simulink model "Multiplier"  (R2019b)
settings: Solver=VariableStepAuto  StartTime=0.0  StopTime=10.0  RelTol=1e-3
libraries: hdlsllib x17
(part 1 of 3)
settings Model: Creator=cohen  LastModifiedBy=cohen

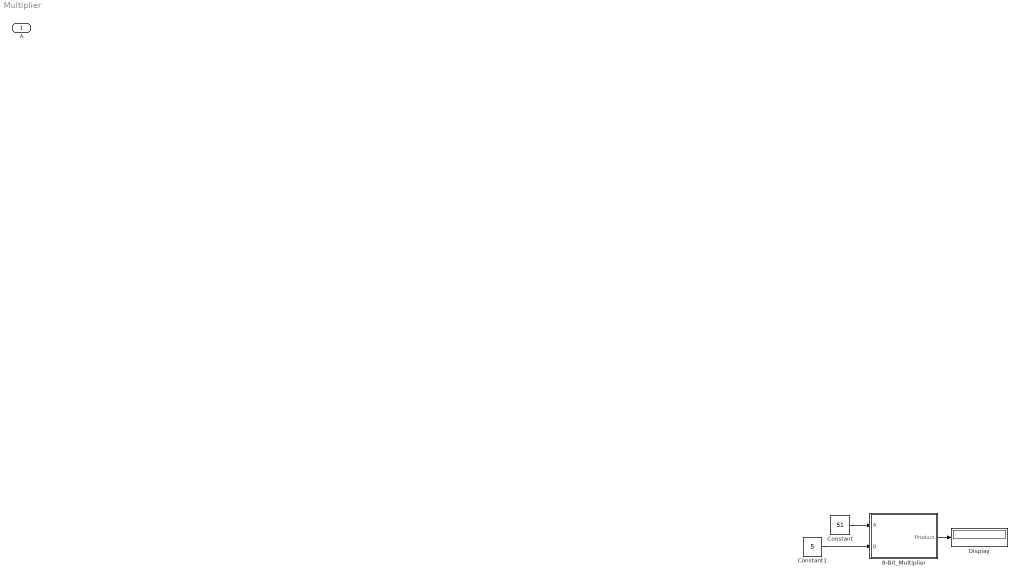
== system Multiplier ==
  A : Inport
  8-Bit_Multiplier : Subsystem
  Constant : Constant  Value=51  OutDataTypeStr=uint8
  Constant1 : Constant  Value=5  OutDataTypeStr=uint8
  Display : Display
  wires:
  8-Bit_Multiplier/1(Product) -> Display/1
  Constant/1 -> 8-Bit_Multiplier/1(A)
  Constant1/1 -> 8-Bit_Multiplier/2(B)

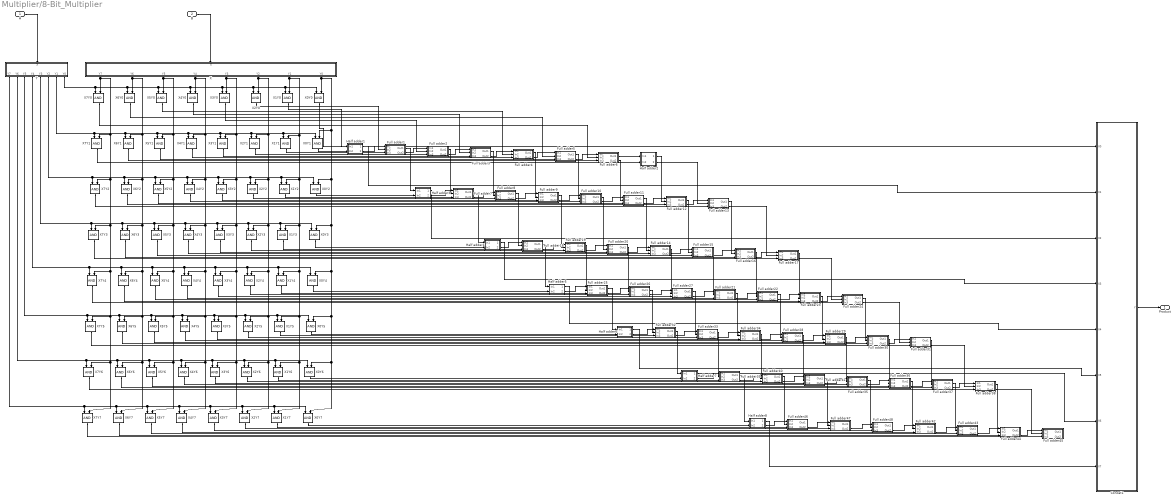
== system Multiplier/8-Bit_Multiplier ==
  A : Inport
  B : Inport  Port=2
  Concat1 : Subsystem
  Full adder1 : Subsystem
  Full adder10 : Subsystem
  Full adder11 : Subsystem
  Full adder12 : Subsystem
  Full adder13 : Subsystem
  Full adder14 : Subsystem
  Full adder15 : Subsystem
  Full adder16 : Subsystem
  Full adder17 : Subsystem
  Full adder18 : Subsystem
  Full adder19 : Subsystem
  Full adder2 : Subsystem
  Full adder20 : Subsystem
  Full adder21 : Subsystem
  Full adder22 : Subsystem
  Full adder23 : Subsystem
  Full adder24 : Subsystem
  Full adder25 : Subsystem
  Full adder26 : Subsystem
  Full adder27 : Subsystem
  Full adder28 : Subsystem
  Full adder29 : Subsystem
  Full adder3 : Subsystem
  Full adder30 : Subsystem
  Full adder31 : Subsystem
  Full adder32 : Subsystem
  Full adder33 : Subsystem
  Full adder34 : Subsystem
  Full adder35 : Subsystem
  Full adder36 : Subsystem
  Full adder37 : Subsystem
  Full adder38 : Subsystem
  Full adder39 : Subsystem
  Full adder4 : Subsystem
  Full adder40 : Subsystem
  Full adder41 : Subsystem
  Full adder42 : Subsystem
  Full adder43 : Subsystem
  Full adder44 : Subsystem
  Full adder45 : Subsystem
  Full adder46 : Subsystem
  Full adder47 : Subsystem
  Full adder48 : Subsystem
  Full adder5 : Subsystem
  Full adder6 : Subsystem
  Full adder7 : Subsystem
  Full adder8 : Subsystem
  Full adder9 : Subsystem
  Half adder1 : Subsystem
  Half adder2 : Subsystem
  Half adder3 : Subsystem
  Half adder4 : Subsystem
  Half adder5 : Subsystem
  Half adder6 : Subsystem
  Half adder7 : Subsystem
  Half adder8 : Subsystem
  X : Subsystem
  X0Y{0..7} (8 alike) : Logic  AllPortsSameDT=off  OutDataTypeStr=boolean
  X1Y{0..7} (8 alike) : Logic  AllPortsSameDT=off  OutDataTypeStr=boolean
  X2Y{0..7} (8 alike) : Logic  AllPortsSameDT=off  OutDataTypeStr=boolean
  X3Y{0..7} (8 alike) : Logic  AllPortsSameDT=off  OutDataTypeStr=boolean
  X4Y{0..7} (8 alike) : Logic  AllPortsSameDT=off  OutDataTypeStr=boolean
  X5Y{0..7} (8 alike) : Logic  AllPortsSameDT=off  OutDataTypeStr=boolean
  X6Y{0..7} (8 alike) : Logic  AllPortsSameDT=off  OutDataTypeStr=boolean
  X7Y{0..7} (8 alike) : Logic  AllPortsSameDT=off  OutDataTypeStr=boolean
  Y : Subsystem
  Product : Outport
  wires:
  X/3(Y5) -> X5Y1/2, X5Y7/2, X5Y6/2, X5Y5/2, X5Y4/2, X5Y3/2, X5Y2/2, X5Y0/2
  Full adder31/2(Out2) -> Full adder38/2(In2)
  Half adder5/1(Out1) -> Concat1/5(X4)
  Full adder4/1(Out1) -> Full adder9/2(In2)
  Full adder15/1(Out1) -> Full adder21/2(In2)
  Full adder10/2(Out2) -> Full adder11/1(In1)
  Full adder3/2(Out2) -> Full adder4/1(In1)
  Full adder7/2(Out2) -> Full adder8/1(In1)
  X/8(Y0) -> X0Y7/2, X0Y6/2, X0Y5/2, X0Y4/2, X0Y3/2, X0Y2/2, X0Y1/2, X0Y0/2
  Full adder21/2(Out2) -> Full adder22/1(In1)
  Full adder5/1(Out1) -> Full adder10/2(In2)
  X/4(Y4) -> X4Y1/2, X4Y7/2, X4Y6/2, X4Y5/2, X4Y4/2, X4Y3/2, X4Y2/2, X4Y0/2
  X6Y4/1 -> Full adder23/3(In3)
  Full adder11/2(Out2) -> Full adder12/1(In1)
  X/5(Y3) -> X3Y1/2, X3Y7/2, X3Y6/2, X3Y5/2, X3Y4/2, X3Y3/2, X3Y2/2, X3Y0/2
  Full adder15/2(Out2) -> Full adder16/1(In1)
  Full adder32/1(Out1) -> Half adder7/1(In1)
  X5Y6/1 -> Full adder36/3(In3)
  Full adder38/2(Out2) -> Full adder45/2(In2)
  Full adder46/2(Out2) -> Full adder47/1(In1)
  Full adder6/2(Out2) -> Full adder11/2(In2)
  X5Y5/1 -> Full adder29/3(In3)
  X/2(Y6) -> X6Y1/2, X6Y7/2, X6Y6/2, X6Y5/2, X6Y4/2, X6Y3/2, X6Y2/2, X6Y0/2
  Full adder44/2(Out2) -> Full adder45/1(In1)
  Half adder4/1(Out1) -> Concat1/4(X3)
  Full adder38/1(Out1) -> Full adder44/2(In2)
  X/1(Y7) -> X7Y1/2, X7Y7/2, X7Y6/2, X7Y5/2, X7Y4/2, X7Y3/2, X7Y2/2, X7Y0/2
  Full adder8/2(Out2) -> Full adder9/1(In1)
  Full adder43/2(Out2) -> Full adder44/1(In1)
  Y/7(Y1) -> X7Y1/1, X6Y1/1, X5Y1/1, X4Y1/1, X3Y1/1, X2Y1/1, X1Y1/1, X0Y1/1
  X/6(Y2) -> X2Y1/2, X2Y7/2, X2Y6/2, X2Y5/2, X2Y4/2, X2Y3/2, X2Y2/2, X2Y0/2
  Half adder8/2(Out2) -> Full adder46/1(In1)
  Full adder13/2(Out2) -> Full adder17/2(In2)
  X1Y1/1 -> Full adder1/3(In3)
  Half adder6/1(Out1) -> Concat1/6(X5)
  Half adder3/2(Out2) -> Full adder7/1(In1)
  X4Y6/1 -> Full adder35/3(In3)
  Full adder11/1(Out1) -> Full adder14/2(In2)
  Full adder27/1(Out1) -> Full adder33/2(In2)
  Full adder42/2(Out2) -> Full adder43/1(In1)
  Y/4(Y4) -> X7Y4/1, X6Y4/1, X5Y4/1, X4Y4/1, X3Y4/1, X2Y4/1, X1Y4/1, X0Y4/1
  Full adder33/2(Out2) -> Full adder34/1(In1)
  Full adder23/1(Out1) -> Full adder29/2(In2)
  X0Y0/1 -> Concat1/1(X0)
  Full adder18/2(Out2) -> Full adder19/1(In1)
  Full adder37/2(Out2) -> Full adder38/1(In1)
  Full adder36/1(Out1) -> Full adder42/2(In2)
  Full adder37/1(Out1) -> Full adder43/2(In2)
  Y/3(Y5) -> X7Y5/1, X6Y5/1, X5Y5/1, X4Y5/1, X3Y5/1, X2Y5/1, X1Y5/1, X0Y5/1
  Half adder3/1(Out1) -> Concat1/3(X2)
  Half adder4/2(Out2) -> Full adder18/1(In1)
  X2Y2/1 -> Full adder8/3(In3)
  X7Y1/1 -> Half adder2/2(In2)
  Full adder17/2(Out2) -> Full adder24/2(In2)
  Y/2(Y6) -> X7Y6/1, X6Y6/1, X5Y6/1, X4Y6/1, X3Y6/1, X2Y6/1, X1Y6/1, X0Y6/1
  Half adder6/2(Out2) -> Full adder32/1(In1)
  Full adder23/2(Out2) -> Full adder24/1(In1)
  Full adder21/1(Out1) -> Full adder34/2(In2)
  X/7(Y1) -> X1Y1/2, X1Y7/2, X1Y6/2, X1Y5/2, X1Y4/2, X1Y3/2, X1Y2/2, X1Y0/2
  Y/6(Y2) -> X7Y2/1, X6Y2/1, X5Y2/1, X4Y2/1, X3Y2/1, X1Y2/1, X0Y2/1, X2Y2/1
  Full adder31/1(Out1) -> Full adder37/2(In2)
  Half adder1/1(Out1) -> Concat1/2(X1)
  X5Y4/1 -> Full adder22/3(In3)
  Full adder8/1(Out1) -> Full adder18/2(In2)
  Full adder40/1(Out1) -> Full adder46/2(In2)
  Half adder2/1(Out1) -> Full adder12/2(In2)
  Full adder19/2(Out2) -> Full adder20/1(In1)
  Y/8(Y0) -> X7Y0/1, X6Y0/1, X5Y0/1, X4Y0/1, X3Y0/1, X2Y0/1, X1Y0/1, X0Y0/1
  Full adder1/2(Out2) -> Full adder2/1(In1)
  Full adder16/1(Out1) -> Full adder22/2(In2)
  Full adder28/2(Out2) -> Full adder29/1(In1)
  Full adder12/2(Out2) -> Full adder13/1(In1)
  Full adder12/1(Out1) -> Full adder15/2(In2)
  Full adder10/1(Out1) -> Full adder20/2(In2)
  Y/5(Y3) -> X7Y3/1, X6Y3/1, X5Y3/1, X4Y3/1, X3Y3/1, X2Y3/1, X1Y3/1, X0Y3/1
  Full adder32/2(Out2) -> Full adder33/1(In1)
  Full adder26/1(Out1) -> Full adder32/2(In2)
  X3Y5/1 -> Full adder34/3(In3)
  Half adder8/1(Out1) -> Concat1/8(X7)
  Full adder26/2(Out2) -> Full adder27/1(In1)
  Full adder9/2(Out2) -> Full adder10/1(In1)
  Half adder7/2(Out2) -> Full adder39/1(In1)
  Full adder24/1(Out1) -> Full adder30/2(In2)
  Full adder41/2(Out2) -> Full adder35/1(In1)
  Full adder3/1(Out1) -> Full adder8/2(In2)
  Full adder39/1(Out1) -> Half adder8/1(In1)
  Full adder35/1(Out1) -> Full adder48/2(In2)
  Full adder5/2(Out2) -> Full adder6/1(In1)
  Full adder9/1(Out1) -> Full adder19/2(In2)
  Full adder35/2(Out2) -> Full adder36/1(In1)
  Full adder40/2(Out2) -> Full adder41/1(In1)
  X1Y5/1 -> Full adder32/3(In3)
  X2Y6/1 -> Full adder40/3(In3)
  Full adder48/2(Out2) -> Full adder42/1(In1)
  Full adder27/2(Out2) -> Full adder21/1(In1)
  Full adder47/2(Out2) -> Full adder48/1(In1)
  X7Y5/1 -> Full adder31/3(In3)
  Full adder28/1(Out1) -> Full adder41/2(In2)
  Full adder20/2(Out2) -> Full adder14/1(In1)
  X6Y3/1 -> Full adder16/3(In3)
  Full adder7/1(Out1) -> Half adder4/1(In1)
  Full adder34/1(Out1) -> Full adder40/2(In2)
  Full adder29/1(Out1) -> Full adder35/2(In2)
  Full adder34/2(Out2) -> Full adder28/1(In1)
  Full adder22/2(Out2) -> Full adder23/1(In1)
  X6Y5/1 -> Full adder30/3(In3)
  Full adder41/1(Out1) -> Full adder47/2(In2)
  Half adder5/2(Out2) -> Full adder25/1(In1)
  B/1 -> X/1(X)
  X1Y3/1 -> Full adder18/3(In3)
  X4Y3/1 -> Full adder14/3(In3)
  Full adder2/2(Out2) -> Full adder3/1(In1)
  Full adder13/1(Out1) -> Full adder16/2(In2)
  Full adder25/2(Out2) -> Full adder26/1(In1)
  X3Y0/1 -> Full adder2/2(In2)
  Full adder33/1(Out1) -> Full adder39/2(In2)
  Full adder18/1(Out1) -> Half adder5/1(In1)
  Full adder29/2(Out2) -> Full adder30/1(In1)
  X5Y1/1 -> Full adder5/3(In3)
  A/1 -> Y/1(X)
  X2Y5/1 -> Full adder33/3(In3)
  Full adder25/1(Out1) -> Half adder6/1(In1)
  X4Y4/1 -> Full adder21/3(In3)
  Full adder30/1(Out1) -> Full adder36/2(In2)
  Full adder24/2(Out2) -> Full adder31/2(In2)
  Concat1/1(Y) -> Product/1
  Full adder39/2(Out2) -> Full adder40/1(In1)
  Full adder36/2(Out2) -> Full adder37/1(In1)
  Half adder2/2(Out2) -> Full adder13/2(In2)
  Half adder7/1(Out1) -> Concat1/7(X6)
  Full adder16/2(Out2) -> Full adder17/1(In1)
  X0Y4/1 -> Half adder5/2(In2)
  Full adder20/1(Out1) -> Full adder26/2(In2)
  X5Y3/1 -> Full adder15/3(In3)
  X2Y0/1 -> Full adder1/2(In2)
  Half adder1/2(Out2) -> Full adder1/1(In1)
  Full adder22/1(Out1) -> Full adder28/2(In2)
  X2Y3/1 -> Full adder19/3(In3)
  Full adder4/2(Out2) -> Full adder5/1(In1)
  X6Y1/1 -> Full adder6/3(In3)
  Full adder14/2(Out2) -> Full adder15/1(In1)
  Full adder1/1(Out1) -> Half adder3/1(In1)
  Full adder2/1(Out1) -> Full adder7/2(In2)
  Full adder30/2(Out2) -> Full adder31/1(In1)
  Full adder14/1(Out1) -> Full adder27/2(In2)
  X7Y7/1 -> Full adder45/3(In3)
  Full adder17/1(Out1) -> Full adder23/2(In2)
  Y/1(Y7) -> X7Y7/1, X6Y7/1, X5Y7/1, X4Y7/1, X3Y7/1, X2Y7/1, X1Y7/1, X0Y7/1
  Full adder19/1(Out1) -> Full adder25/2(In2)
  X2Y7/1 -> Full adder47/3(In3)
  X2Y4/1 -> Full adder26/3(In3)
  X0Y1/1 -> Half adder1/2(In2)
  X5Y7/1 -> Full adder43/3(In3)
  X5Y2/1 -> Full adder11/3(In3)
  X1Y2/1 -> Full adder7/3(In3)
  X1Y0/1 -> Half adder1/1(In1)
  X0Y3/1 -> Half adder4/2(In2)
  X4Y1/1 -> Full adder4/3(In3)
  X1Y7/1 -> Full adder46/3(In3)
  X7Y4/1 -> Full adder24/3(In3)
  X4Y0/1 -> Full adder3/2(In2)
  X3Y1/1 -> Full adder3/3(In3)
  X3Y3/1 -> Full adder20/3(In3)
  X7Y0/1 -> Full adder6/2(In2)
  X1Y6/1 -> Full adder39/3(In3)
  Full adder6/1(Out1) -> Half adder2/1(In1)
  X5Y0/1 -> Full adder4/2(In2)
  X6Y7/1 -> Full adder44/3(In3)
  X1Y4/1 -> Full adder25/3(In3)
  X0Y2/1 -> Half adder3/2(In2)
  X7Y3/1 -> Full adder17/3(In3)
  X4Y2/1 -> Full adder10/3(In3)
  X7Y2/1 -> Full adder13/3(In3)
  X3Y2/1 -> Full adder9/3(In3)
  X6Y2/1 -> Full adder12/3(In3)
  X3Y4/1 -> Full adder27/3(In3)
  X7Y6/1 -> Full adder38/3(In3)
  X0Y5/1 -> Half adder6/2(In2)
  X4Y5/1 -> Full adder28/3(In3)
  X6Y0/1 -> Full adder5/2(In2)
  X0Y6/1 -> Half adder7/2(In2)
  X4Y7/1 -> Full adder42/3(In3)
  X2Y1/1 -> Full adder2/3(In3)
  X3Y7/1 -> Full adder48/3(In3)
  X6Y6/1 -> Full adder37/3(In3)
  X0Y7/1 -> Half adder8/2(In2)
  X3Y6/1 -> Full adder41/3(In3)

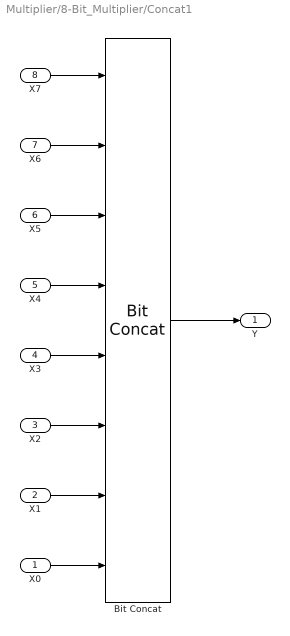
== system Multiplier/8-Bit_Multiplier/Concat1 ==
  X0 : Inport  OutDataTypeStr=boolean  SampleTime=1
  X1 : Inport  Port=2  OutDataTypeStr=boolean  SampleTime=1
  X2 : Inport  Port=3  OutDataTypeStr=boolean  SampleTime=1
  X3 : Inport  Port=4  OutDataTypeStr=boolean  SampleTime=1
  X4 : Inport  Port=5  OutDataTypeStr=boolean  SampleTime=1
  X5 : Inport  Port=6  OutDataTypeStr=boolean  SampleTime=1
  X6 : Inport  Port=7  OutDataTypeStr=boolean  SampleTime=1
  X7 : Inport  Port=8  OutDataTypeStr=boolean  SampleTime=1
  Bit Concat : hdlsllib/Logic and Bit Operations/Bit Concat  numInputs=8
      settings: SourceProductName=Simulink
  Y : Outport
  wires:
  X6/1 -> Bit Concat/2
  X2/1 -> Bit Concat/6
  X7/1 -> Bit Concat/1
  X0/1 -> Bit Concat/8
  Bit Concat/1 -> Y/1
  X3/1 -> Bit Concat/5
  X1/1 -> Bit Concat/7
  X5/1 -> Bit Concat/3
  X4/1 -> Bit Concat/4

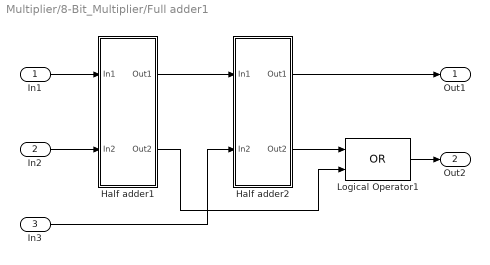
== system Multiplier/8-Bit_Multiplier/Full adder1 ==
  In1 : Inport  OutDataTypeStr=boolean
  In2 : Inport  Port=2  OutDataTypeStr=boolean
  In3 : Inport  Port=3  OutDataTypeStr=boolean
  Half adder1 : Subsystem
  Half adder2 : Subsystem
  Logical Operator1 : Logic  Operator=OR  AllPortsSameDT=off  OutDataTypeStr=boolean
  Out1 : Outport
  Out2 : Outport  Port=2
  wires:
  Logical Operator1/1 -> Out2/1
  In1/1 -> Half adder1/1(In1)
  Half adder2/1(Out1) -> Out1/1
  In2/1 -> Half adder1/2(In2)
  In3/1 -> Half adder2/2(In2)
  Half adder1/2(Out2) -> Logical Operator1/2
  Half adder1/1(Out1) -> Half adder2/1(In1)
  Half adder2/2(Out2) -> Logical Operator1/1

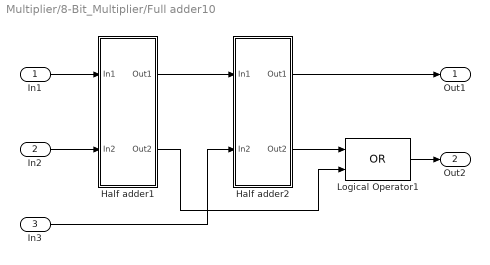
== system Multiplier/8-Bit_Multiplier/Full adder10 ==
  In1 : Inport  OutDataTypeStr=boolean
  In2 : Inport  Port=2  OutDataTypeStr=boolean
  In3 : Inport  Port=3  OutDataTypeStr=boolean
  Half adder1 : Subsystem
  Half adder2 : Subsystem
  Logical Operator1 : Logic  Operator=OR  AllPortsSameDT=off  OutDataTypeStr=boolean
  Out1 : Outport
  Out2 : Outport  Port=2
  wires:
  Logical Operator1/1 -> Out2/1
  In1/1 -> Half adder1/1(In1)
  Half adder2/1(Out1) -> Out1/1
  In2/1 -> Half adder1/2(In2)
  In3/1 -> Half adder2/2(In2)
  Half adder1/2(Out2) -> Logical Operator1/2
  Half adder1/1(Out1) -> Half adder2/1(In1)
  Half adder2/2(Out2) -> Logical Operator1/1

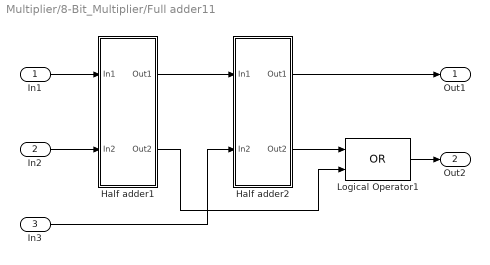
== system Multiplier/8-Bit_Multiplier/Full adder11 ==
  In1 : Inport  OutDataTypeStr=boolean
  In2 : Inport  Port=2  OutDataTypeStr=boolean
  In3 : Inport  Port=3  OutDataTypeStr=boolean
  Half adder1 : Subsystem
  Half adder2 : Subsystem
  Logical Operator1 : Logic  Operator=OR  AllPortsSameDT=off  OutDataTypeStr=boolean
  Out1 : Outport
  Out2 : Outport  Port=2
  wires:
  Logical Operator1/1 -> Out2/1
  In1/1 -> Half adder1/1(In1)
  Half adder2/1(Out1) -> Out1/1
  In2/1 -> Half adder1/2(In2)
  In3/1 -> Half adder2/2(In2)
  Half adder1/2(Out2) -> Logical Operator1/2
  Half adder1/1(Out1) -> Half adder2/1(In1)
  Half adder2/2(Out2) -> Logical Operator1/1

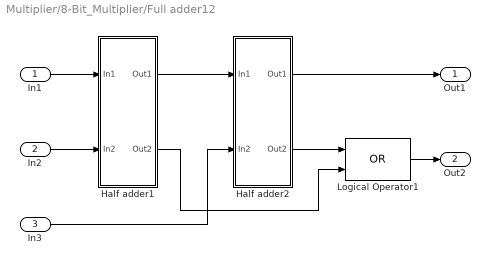
== system Multiplier/8-Bit_Multiplier/Full adder12 ==
  In1 : Inport  OutDataTypeStr=boolean
  In2 : Inport  Port=2  OutDataTypeStr=boolean
  In3 : Inport  Port=3  OutDataTypeStr=boolean
  Half adder1 : Subsystem
  Half adder2 : Subsystem
  Logical Operator1 : Logic  Operator=OR  AllPortsSameDT=off  OutDataTypeStr=boolean
  Out1 : Outport
  Out2 : Outport  Port=2
  wires:
  Logical Operator1/1 -> Out2/1
  In1/1 -> Half adder1/1(In1)
  Half adder2/1(Out1) -> Out1/1
  In2/1 -> Half adder1/2(In2)
  In3/1 -> Half adder2/2(In2)
  Half adder1/2(Out2) -> Logical Operator1/2
  Half adder1/1(Out1) -> Half adder2/1(In1)
  Half adder2/2(Out2) -> Logical Operator1/1

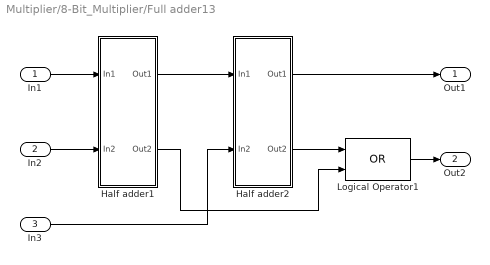
== system Multiplier/8-Bit_Multiplier/Full adder13 ==
  In1 : Inport  OutDataTypeStr=boolean
  In2 : Inport  Port=2  OutDataTypeStr=boolean
  In3 : Inport  Port=3  OutDataTypeStr=boolean
  Half adder1 : Subsystem
  Half adder2 : Subsystem
  Logical Operator1 : Logic  Operator=OR  AllPortsSameDT=off  OutDataTypeStr=boolean
  Out1 : Outport
  Out2 : Outport  Port=2
  wires:
  Logical Operator1/1 -> Out2/1
  In1/1 -> Half adder1/1(In1)
  Half adder2/1(Out1) -> Out1/1
  In2/1 -> Half adder1/2(In2)
  In3/1 -> Half adder2/2(In2)
  Half adder1/2(Out2) -> Logical Operator1/2
  Half adder1/1(Out1) -> Half adder2/1(In1)
  Half adder2/2(Out2) -> Logical Operator1/1

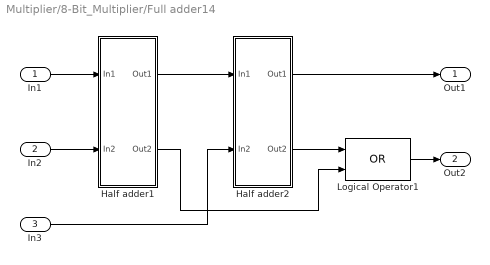
== system Multiplier/8-Bit_Multiplier/Full adder14 ==
  In1 : Inport  OutDataTypeStr=boolean
  In2 : Inport  Port=2  OutDataTypeStr=boolean
  In3 : Inport  Port=3  OutDataTypeStr=boolean
  Half adder1 : Subsystem
  Half adder2 : Subsystem
  Logical Operator1 : Logic  Operator=OR  AllPortsSameDT=off  OutDataTypeStr=boolean
  Out1 : Outport
  Out2 : Outport  Port=2
  wires:
  Logical Operator1/1 -> Out2/1
  In1/1 -> Half adder1/1(In1)
  Half adder2/1(Out1) -> Out1/1
  In2/1 -> Half adder1/2(In2)
  In3/1 -> Half adder2/2(In2)
  Half adder1/2(Out2) -> Logical Operator1/2
  Half adder1/1(Out1) -> Half adder2/1(In1)
  Half adder2/2(Out2) -> Logical Operator1/1

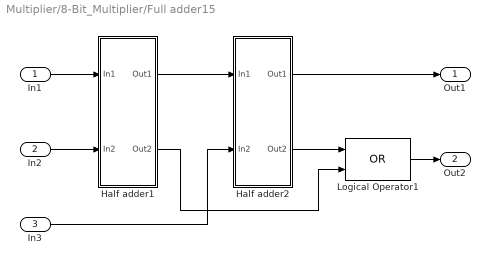
== system Multiplier/8-Bit_Multiplier/Full adder15 ==
  In1 : Inport  OutDataTypeStr=boolean
  In2 : Inport  Port=2  OutDataTypeStr=boolean
  In3 : Inport  Port=3  OutDataTypeStr=boolean
  Half adder1 : Subsystem
  Half adder2 : Subsystem
  Logical Operator1 : Logic  Operator=OR  AllPortsSameDT=off  OutDataTypeStr=boolean
  Out1 : Outport
  Out2 : Outport  Port=2
  wires:
  Logical Operator1/1 -> Out2/1
  In1/1 -> Half adder1/1(In1)
  Half adder2/1(Out1) -> Out1/1
  In2/1 -> Half adder1/2(In2)
  In3/1 -> Half adder2/2(In2)
  Half adder1/2(Out2) -> Logical Operator1/2
  Half adder1/1(Out1) -> Half adder2/1(In1)
  Half adder2/2(Out2) -> Logical Operator1/1

== system Multiplier/8-Bit_Multiplier/Full adder16 ==
  In1 : Inport  OutDataTypeStr=boolean
  In2 : Inport  Port=2  OutDataTypeStr=boolean
  In3 : Inport  Port=3  OutDataTypeStr=boolean
  Half adder1 : Subsystem
  Half adder2 : Subsystem
  Logical Operator1 : Logic  Operator=OR  AllPortsSameDT=off  OutDataTypeStr=boolean
  Out1 : Outport
  Out2 : Outport  Port=2
  wires:
  Logical Operator1/1 -> Out2/1
  In1/1 -> Half adder1/1(In1)
  Half adder2/1(Out1) -> Out1/1
  In2/1 -> Half adder1/2(In2)
  In3/1 -> Half adder2/2(In2)
  Half adder1/2(Out2) -> Logical Operator1/2
  Half adder1/1(Out1) -> Half adder2/1(In1)
  Half adder2/2(Out2) -> Logical Operator1/1

== system Multiplier/8-Bit_Multiplier/Full adder17 ==
  In1 : Inport  OutDataTypeStr=boolean
  In2 : Inport  Port=2  OutDataTypeStr=boolean
  In3 : Inport  Port=3  OutDataTypeStr=boolean
  Half adder1 : Subsystem
  Half adder2 : Subsystem
  Logical Operator1 : Logic  Operator=OR  AllPortsSameDT=off  OutDataTypeStr=boolean
  Out1 : Outport
  Out2 : Outport  Port=2
  wires:
  Logical Operator1/1 -> Out2/1
  In1/1 -> Half adder1/1(In1)
  Half adder2/1(Out1) -> Out1/1
  In2/1 -> Half adder1/2(In2)
  In3/1 -> Half adder2/2(In2)
  Half adder1/2(Out2) -> Logical Operator1/2
  Half adder1/1(Out1) -> Half adder2/1(In1)
  Half adder2/2(Out2) -> Logical Operator1/1

== system Multiplier/8-Bit_Multiplier/Full adder18 ==
  In1 : Inport  OutDataTypeStr=boolean
  In2 : Inport  Port=2  OutDataTypeStr=boolean
  In3 : Inport  Port=3  OutDataTypeStr=boolean
  Half adder1 : Subsystem
  Half adder2 : Subsystem
  Logical Operator1 : Logic  Operator=OR  AllPortsSameDT=off  OutDataTypeStr=boolean
  Out1 : Outport
  Out2 : Outport  Port=2
  wires:
  Logical Operator1/1 -> Out2/1
  In1/1 -> Half adder1/1(In1)
  Half adder2/1(Out1) -> Out1/1
  In2/1 -> Half adder1/2(In2)
  In3/1 -> Half adder2/2(In2)
  Half adder1/2(Out2) -> Logical Operator1/2
  Half adder1/1(Out1) -> Half adder2/1(In1)
  Half adder2/2(Out2) -> Logical Operator1/1

== system Multiplier/8-Bit_Multiplier/Full adder19 ==
  In1 : Inport  OutDataTypeStr=boolean
  In2 : Inport  Port=2  OutDataTypeStr=boolean
  In3 : Inport  Port=3  OutDataTypeStr=boolean
  Half adder1 : Subsystem
  Half adder2 : Subsystem
  Logical Operator1 : Logic  Operator=OR  AllPortsSameDT=off  OutDataTypeStr=boolean
  Out1 : Outport
  Out2 : Outport  Port=2
  wires:
  Logical Operator1/1 -> Out2/1
  In1/1 -> Half adder1/1(In1)
  Half adder2/1(Out1) -> Out1/1
  In2/1 -> Half adder1/2(In2)
  In3/1 -> Half adder2/2(In2)
  Half adder1/2(Out2) -> Logical Operator1/2
  Half adder1/1(Out1) -> Half adder2/1(In1)
  Half adder2/2(Out2) -> Logical Operator1/1

== system Multiplier/8-Bit_Multiplier/Full adder2 ==
  In1 : Inport  OutDataTypeStr=boolean
  In2 : Inport  Port=2  OutDataTypeStr=boolean
  In3 : Inport  Port=3  OutDataTypeStr=boolean
  Half adder1 : Subsystem
  Half adder2 : Subsystem
  Logical Operator1 : Logic  Operator=OR  AllPortsSameDT=off  OutDataTypeStr=boolean
  Out1 : Outport
  Out2 : Outport  Port=2
  wires:
  Logical Operator1/1 -> Out2/1
  In1/1 -> Half adder1/1(In1)
  Half adder2/1(Out1) -> Out1/1
  In2/1 -> Half adder1/2(In2)
  In3/1 -> Half adder2/2(In2)
  Half adder1/2(Out2) -> Logical Operator1/2
  Half adder1/1(Out1) -> Half adder2/1(In1)
  Half adder2/2(Out2) -> Logical Operator1/1

== system Multiplier/8-Bit_Multiplier/Full adder20 ==
  In1 : Inport  OutDataTypeStr=boolean
  In2 : Inport  Port=2  OutDataTypeStr=boolean
  In3 : Inport  Port=3  OutDataTypeStr=boolean
  Half adder1 : Subsystem
  Half adder2 : Subsystem
  Logical Operator1 : Logic  Operator=OR  AllPortsSameDT=off  OutDataTypeStr=boolean
  Out1 : Outport
  Out2 : Outport  Port=2
  wires:
  Logical Operator1/1 -> Out2/1
  In1/1 -> Half adder1/1(In1)
  Half adder2/1(Out1) -> Out1/1
  In2/1 -> Half adder1/2(In2)
  In3/1 -> Half adder2/2(In2)
  Half adder1/2(Out2) -> Logical Operator1/2
  Half adder1/1(Out1) -> Half adder2/1(In1)
  Half adder2/2(Out2) -> Logical Operator1/1

== system Multiplier/8-Bit_Multiplier/Full adder21 ==
  In1 : Inport  OutDataTypeStr=boolean
  In2 : Inport  Port=2  OutDataTypeStr=boolean
  In3 : Inport  Port=3  OutDataTypeStr=boolean
  Half adder1 : Subsystem
  Half adder2 : Subsystem
  Logical Operator1 : Logic  Operator=OR  AllPortsSameDT=off  OutDataTypeStr=boolean
  Out1 : Outport
  Out2 : Outport  Port=2
  wires:
  Logical Operator1/1 -> Out2/1
  In1/1 -> Half adder1/1(In1)
  Half adder2/1(Out1) -> Out1/1
  In2/1 -> Half adder1/2(In2)
  In3/1 -> Half adder2/2(In2)
  Half adder1/2(Out2) -> Logical Operator1/2
  Half adder1/1(Out1) -> Half adder2/1(In1)
  Half adder2/2(Out2) -> Logical Operator1/1

== system Multiplier/8-Bit_Multiplier/Full adder22 ==
  In1 : Inport  OutDataTypeStr=boolean
  In2 : Inport  Port=2  OutDataTypeStr=boolean
  In3 : Inport  Port=3  OutDataTypeStr=boolean
  Half adder1 : Subsystem
  Half adder2 : Subsystem
  Logical Operator1 : Logic  Operator=OR  AllPortsSameDT=off  OutDataTypeStr=boolean
  Out1 : Outport
  Out2 : Outport  Port=2
  wires:
  Logical Operator1/1 -> Out2/1
  In1/1 -> Half adder1/1(In1)
  Half adder2/1(Out1) -> Out1/1
  In2/1 -> Half adder1/2(In2)
  In3/1 -> Half adder2/2(In2)
  Half adder1/2(Out2) -> Logical Operator1/2
  Half adder1/1(Out1) -> Half adder2/1(In1)
  Half adder2/2(Out2) -> Logical Operator1/1

== system Multiplier/8-Bit_Multiplier/Full adder23 ==
  In1 : Inport  OutDataTypeStr=boolean
  In2 : Inport  Port=2  OutDataTypeStr=boolean
  In3 : Inport  Port=3  OutDataTypeStr=boolean
  Half adder1 : Subsystem
  Half adder2 : Subsystem
  Logical Operator1 : Logic  Operator=OR  AllPortsSameDT=off  OutDataTypeStr=boolean
  Out1 : Outport
  Out2 : Outport  Port=2
  wires:
  Logical Operator1/1 -> Out2/1
  In1/1 -> Half adder1/1(In1)
  Half adder2/1(Out1) -> Out1/1
  In2/1 -> Half adder1/2(In2)
  In3/1 -> Half adder2/2(In2)
  Half adder1/2(Out2) -> Logical Operator1/2
  Half adder1/1(Out1) -> Half adder2/1(In1)
  Half adder2/2(Out2) -> Logical Operator1/1

== system Multiplier/8-Bit_Multiplier/Full adder24 ==
  In1 : Inport  OutDataTypeStr=boolean
  In2 : Inport  Port=2  OutDataTypeStr=boolean
  In3 : Inport  Port=3  OutDataTypeStr=boolean
  Half adder1 : Subsystem
  Half adder2 : Subsystem
  Logical Operator1 : Logic  Operator=OR  AllPortsSameDT=off  OutDataTypeStr=boolean
  Out1 : Outport
  Out2 : Outport  Port=2
  wires:
  Logical Operator1/1 -> Out2/1
  In1/1 -> Half adder1/1(In1)
  Half adder2/1(Out1) -> Out1/1
  In2/1 -> Half adder1/2(In2)
  In3/1 -> Half adder2/2(In2)
  Half adder1/2(Out2) -> Logical Operator1/2
  Half adder1/1(Out1) -> Half adder2/1(In1)
  Half adder2/2(Out2) -> Logical Operator1/1

== system Multiplier/8-Bit_Multiplier/Full adder25 ==
  In1 : Inport  OutDataTypeStr=boolean
  In2 : Inport  Port=2  OutDataTypeStr=boolean
  In3 : Inport  Port=3  OutDataTypeStr=boolean
  Half adder1 : Subsystem
  Half adder2 : Subsystem
  Logical Operator1 : Logic  Operator=OR  AllPortsSameDT=off  OutDataTypeStr=boolean
  Out1 : Outport
  Out2 : Outport  Port=2
  wires:
  Logical Operator1/1 -> Out2/1
  In1/1 -> Half adder1/1(In1)
  Half adder2/1(Out1) -> Out1/1
  In2/1 -> Half adder1/2(In2)
  In3/1 -> Half adder2/2(In2)
  Half adder1/2(Out2) -> Logical Operator1/2
  Half adder1/1(Out1) -> Half adder2/1(In1)
  Half adder2/2(Out2) -> Logical Operator1/1

== system Multiplier/8-Bit_Multiplier/Full adder26 ==
  In1 : Inport  OutDataTypeStr=boolean
  In2 : Inport  Port=2  OutDataTypeStr=boolean
  In3 : Inport  Port=3  OutDataTypeStr=boolean
  Half adder1 : Subsystem
  Half adder2 : Subsystem
  Logical Operator1 : Logic  Operator=OR  AllPortsSameDT=off  OutDataTypeStr=boolean
  Out1 : Outport
  Out2 : Outport  Port=2
  wires:
  Logical Operator1/1 -> Out2/1
  In1/1 -> Half adder1/1(In1)
  Half adder2/1(Out1) -> Out1/1
  In2/1 -> Half adder1/2(In2)
  In3/1 -> Half adder2/2(In2)
  Half adder1/2(Out2) -> Logical Operator1/2
  Half adder1/1(Out1) -> Half adder2/1(In1)
  Half adder2/2(Out2) -> Logical Operator1/1

== system Multiplier/8-Bit_Multiplier/Full adder27 ==
  In1 : Inport  OutDataTypeStr=boolean
  In2 : Inport  Port=2  OutDataTypeStr=boolean
  In3 : Inport  Port=3  OutDataTypeStr=boolean
  Half adder1 : Subsystem
  Half adder2 : Subsystem
  Logical Operator1 : Logic  Operator=OR  AllPortsSameDT=off  OutDataTypeStr=boolean
  Out1 : Outport
  Out2 : Outport  Port=2
  wires:
  Logical Operator1/1 -> Out2/1
  In1/1 -> Half adder1/1(In1)
  Half adder2/1(Out1) -> Out1/1
  In2/1 -> Half adder1/2(In2)
  In3/1 -> Half adder2/2(In2)
  Half adder1/2(Out2) -> Logical Operator1/2
  Half adder1/1(Out1) -> Half adder2/1(In1)
  Half adder2/2(Out2) -> Logical Operator1/1

== system Multiplier/8-Bit_Multiplier/Full adder28 ==
  In1 : Inport  OutDataTypeStr=boolean
  In2 : Inport  Port=2  OutDataTypeStr=boolean
  In3 : Inport  Port=3  OutDataTypeStr=boolean
  Half adder1 : Subsystem
  Half adder2 : Subsystem
  Logical Operator1 : Logic  Operator=OR  AllPortsSameDT=off  OutDataTypeStr=boolean
  Out1 : Outport
  Out2 : Outport  Port=2
  wires:
  Logical Operator1/1 -> Out2/1
  In1/1 -> Half adder1/1(In1)
  Half adder2/1(Out1) -> Out1/1
  In2/1 -> Half adder1/2(In2)
  In3/1 -> Half adder2/2(In2)
  Half adder1/2(Out2) -> Logical Operator1/2
  Half adder1/1(Out1) -> Half adder2/1(In1)
  Half adder2/2(Out2) -> Logical Operator1/1

== system Multiplier/8-Bit_Multiplier/Full adder29 ==
  In1 : Inport  OutDataTypeStr=boolean
  In2 : Inport  Port=2  OutDataTypeStr=boolean
  In3 : Inport  Port=3  OutDataTypeStr=boolean
  Half adder1 : Subsystem
  Half adder2 : Subsystem
  Logical Operator1 : Logic  Operator=OR  AllPortsSameDT=off  OutDataTypeStr=boolean
  Out1 : Outport
  Out2 : Outport  Port=2
  wires:
  Logical Operator1/1 -> Out2/1
  In1/1 -> Half adder1/1(In1)
  Half adder2/1(Out1) -> Out1/1
  In2/1 -> Half adder1/2(In2)
  In3/1 -> Half adder2/2(In2)
  Half adder1/2(Out2) -> Logical Operator1/2
  Half adder1/1(Out1) -> Half adder2/1(In1)
  Half adder2/2(Out2) -> Logical Operator1/1

== system Multiplier/8-Bit_Multiplier/Full adder3 ==
  In1 : Inport  OutDataTypeStr=boolean
  In2 : Inport  Port=2  OutDataTypeStr=boolean
  In3 : Inport  Port=3  OutDataTypeStr=boolean
  Half adder1 : Subsystem
  Half adder2 : Subsystem
  Logical Operator1 : Logic  Operator=OR  AllPortsSameDT=off  OutDataTypeStr=boolean
  Out1 : Outport
  Out2 : Outport  Port=2
  wires:
  Logical Operator1/1 -> Out2/1
  In1/1 -> Half adder1/1(In1)
  Half adder2/1(Out1) -> Out1/1
  In2/1 -> Half adder1/2(In2)
  In3/1 -> Half adder2/2(In2)
  Half adder1/2(Out2) -> Logical Operator1/2
  Half adder1/1(Out1) -> Half adder2/1(In1)
  Half adder2/2(Out2) -> Logical Operator1/1

== system Multiplier/8-Bit_Multiplier/Full adder30 ==
  In1 : Inport  OutDataTypeStr=boolean
  In2 : Inport  Port=2  OutDataTypeStr=boolean
  In3 : Inport  Port=3  OutDataTypeStr=boolean
  Half adder1 : Subsystem
  Half adder2 : Subsystem
  Logical Operator1 : Logic  Operator=OR  AllPortsSameDT=off  OutDataTypeStr=boolean
  Out1 : Outport
  Out2 : Outport  Port=2
  wires:
  Logical Operator1/1 -> Out2/1
  In1/1 -> Half adder1/1(In1)
  Half adder2/1(Out1) -> Out1/1
  In2/1 -> Half adder1/2(In2)
  In3/1 -> Half adder2/2(In2)
  Half adder1/2(Out2) -> Logical Operator1/2
  Half adder1/1(Out1) -> Half adder2/1(In1)
  Half adder2/2(Out2) -> Logical Operator1/1

== system Multiplier/8-Bit_Multiplier/Full adder31 ==
  In1 : Inport  OutDataTypeStr=boolean
  In2 : Inport  Port=2  OutDataTypeStr=boolean
  In3 : Inport  Port=3  OutDataTypeStr=boolean
  Half adder1 : Subsystem
  Half adder2 : Subsystem
  Logical Operator1 : Logic  Operator=OR  AllPortsSameDT=off  OutDataTypeStr=boolean
  Out1 : Outport
  Out2 : Outport  Port=2
  wires:
  Logical Operator1/1 -> Out2/1
  In1/1 -> Half adder1/1(In1)
  Half adder2/1(Out1) -> Out1/1
  In2/1 -> Half adder1/2(In2)
  In3/1 -> Half adder2/2(In2)
  Half adder1/2(Out2) -> Logical Operator1/2
  Half adder1/1(Out1) -> Half adder2/1(In1)
  Half adder2/2(Out2) -> Logical Operator1/1

== system Multiplier/8-Bit_Multiplier/Full adder32 ==
  In1 : Inport  OutDataTypeStr=boolean
  In2 : Inport  Port=2  OutDataTypeStr=boolean
  In3 : Inport  Port=3  OutDataTypeStr=boolean
  Half adder1 : Subsystem
  Half adder2 : Subsystem
  Logical Operator1 : Logic  Operator=OR  AllPortsSameDT=off  OutDataTypeStr=boolean
  Out1 : Outport
  Out2 : Outport  Port=2
  wires:
  Logical Operator1/1 -> Out2/1
  In1/1 -> Half adder1/1(In1)
  Half adder2/1(Out1) -> Out1/1
  In2/1 -> Half adder1/2(In2)
  In3/1 -> Half adder2/2(In2)
  Half adder1/2(Out2) -> Logical Operator1/2
  Half adder1/1(Out1) -> Half adder2/1(In1)
  Half adder2/2(Out2) -> Logical Operator1/1

== system Multiplier/8-Bit_Multiplier/Full adder33 ==
  In1 : Inport  OutDataTypeStr=boolean
  In2 : Inport  Port=2  OutDataTypeStr=boolean
  In3 : Inport  Port=3  OutDataTypeStr=boolean
  Half adder1 : Subsystem
  Half adder2 : Subsystem
  Logical Operator1 : Logic  Operator=OR  AllPortsSameDT=off  OutDataTypeStr=boolean
  Out1 : Outport
  Out2 : Outport  Port=2
  wires:
  Logical Operator1/1 -> Out2/1
  In1/1 -> Half adder1/1(In1)
  Half adder2/1(Out1) -> Out1/1
  In2/1 -> Half adder1/2(In2)
  In3/1 -> Half adder2/2(In2)
  Half adder1/2(Out2) -> Logical Operator1/2
  Half adder1/1(Out1) -> Half adder2/1(In1)
  Half adder2/2(Out2) -> Logical Operator1/1

== system Multiplier/8-Bit_Multiplier/Full adder34 ==
  In1 : Inport  OutDataTypeStr=boolean
  In2 : Inport  Port=2  OutDataTypeStr=boolean
  In3 : Inport  Port=3  OutDataTypeStr=boolean
  Half adder1 : Subsystem
  Half adder2 : Subsystem
  Logical Operator1 : Logic  Operator=OR  AllPortsSameDT=off  OutDataTypeStr=boolean
  Out1 : Outport
  Out2 : Outport  Port=2
  wires:
  Logical Operator1/1 -> Out2/1
  In1/1 -> Half adder1/1(In1)
  Half adder2/1(Out1) -> Out1/1
  In2/1 -> Half adder1/2(In2)
  In3/1 -> Half adder2/2(In2)
  Half adder1/2(Out2) -> Logical Operator1/2
  Half adder1/1(Out1) -> Half adder2/1(In1)
  Half adder2/2(Out2) -> Logical Operator1/1

== system Multiplier/8-Bit_Multiplier/Full adder35 ==
  In1 : Inport  OutDataTypeStr=boolean
  In2 : Inport  Port=2  OutDataTypeStr=boolean
  In3 : Inport  Port=3  OutDataTypeStr=boolean
  Half adder1 : Subsystem
  Half adder2 : Subsystem
  Logical Operator1 : Logic  Operator=OR  AllPortsSameDT=off  OutDataTypeStr=boolean
  Out1 : Outport
  Out2 : Outport  Port=2
  wires:
  Logical Operator1/1 -> Out2/1
  In1/1 -> Half adder1/1(In1)
  Half adder2/1(Out1) -> Out1/1
  In2/1 -> Half adder1/2(In2)
  In3/1 -> Half adder2/2(In2)
  Half adder1/2(Out2) -> Logical Operator1/2
  Half adder1/1(Out1) -> Half adder2/1(In1)
  Half adder2/2(Out2) -> Logical Operator1/1

== system Multiplier/8-Bit_Multiplier/Full adder36 ==
  In1 : Inport  OutDataTypeStr=boolean
  In2 : Inport  Port=2  OutDataTypeStr=boolean
  In3 : Inport  Port=3  OutDataTypeStr=boolean
  Half adder1 : Subsystem
  Half adder2 : Subsystem
  Logical Operator1 : Logic  Operator=OR  AllPortsSameDT=off  OutDataTypeStr=boolean
  Out1 : Outport
  Out2 : Outport  Port=2
  wires:
  Logical Operator1/1 -> Out2/1
  In1/1 -> Half adder1/1(In1)
  Half adder2/1(Out1) -> Out1/1
  In2/1 -> Half adder1/2(In2)
  In3/1 -> Half adder2/2(In2)
  Half adder1/2(Out2) -> Logical Operator1/2
  Half adder1/1(Out1) -> Half adder2/1(In1)
  Half adder2/2(Out2) -> Logical Operator1/1

== system Multiplier/8-Bit_Multiplier/Full adder37 ==
  In1 : Inport  OutDataTypeStr=boolean
  In2 : Inport  Port=2  OutDataTypeStr=boolean
  In3 : Inport  Port=3  OutDataTypeStr=boolean
  Half adder1 : Subsystem
  Half adder2 : Subsystem
  Logical Operator1 : Logic  Operator=OR  AllPortsSameDT=off  OutDataTypeStr=boolean
  Out1 : Outport
  Out2 : Outport  Port=2
  wires:
  Logical Operator1/1 -> Out2/1
  In1/1 -> Half adder1/1(In1)
  Half adder2/1(Out1) -> Out1/1
  In2/1 -> Half adder1/2(In2)
  In3/1 -> Half adder2/2(In2)
  Half adder1/2(Out2) -> Logical Operator1/2
  Half adder1/1(Out1) -> Half adder2/1(In1)
  Half adder2/2(Out2) -> Logical Operator1/1

== system Multiplier/8-Bit_Multiplier/Full adder38 ==
  In1 : Inport  OutDataTypeStr=boolean
  In2 : Inport  Port=2  OutDataTypeStr=boolean
  In3 : Inport  Port=3  OutDataTypeStr=boolean
  Half adder1 : Subsystem
  Half adder2 : Subsystem
  Logical Operator1 : Logic  Operator=OR  AllPortsSameDT=off  OutDataTypeStr=boolean
  Out1 : Outport
  Out2 : Outport  Port=2
  wires:
  Logical Operator1/1 -> Out2/1
  In1/1 -> Half adder1/1(In1)
  Half adder2/1(Out1) -> Out1/1
  In2/1 -> Half adder1/2(In2)
  In3/1 -> Half adder2/2(In2)
  Half adder1/2(Out2) -> Logical Operator1/2
  Half adder1/1(Out1) -> Half adder2/1(In1)
  Half adder2/2(Out2) -> Logical Operator1/1

== system Multiplier/8-Bit_Multiplier/Full adder39 ==
  In1 : Inport  OutDataTypeStr=boolean
  In2 : Inport  Port=2  OutDataTypeStr=boolean
  In3 : Inport  Port=3  OutDataTypeStr=boolean
  Half adder1 : Subsystem
  Half adder2 : Subsystem
  Logical Operator1 : Logic  Operator=OR  AllPortsSameDT=off  OutDataTypeStr=boolean
  Out1 : Outport
  Out2 : Outport  Port=2
  wires:
  Logical Operator1/1 -> Out2/1
  In1/1 -> Half adder1/1(In1)
  Half adder2/1(Out1) -> Out1/1
  In2/1 -> Half adder1/2(In2)
  In3/1 -> Half adder2/2(In2)
  Half adder1/2(Out2) -> Logical Operator1/2
  Half adder1/1(Out1) -> Half adder2/1(In1)
  Half adder2/2(Out2) -> Logical Operator1/1

== system Multiplier/8-Bit_Multiplier/Full adder4 ==
  In1 : Inport  OutDataTypeStr=boolean
  In2 : Inport  Port=2  OutDataTypeStr=boolean
  In3 : Inport  Port=3  OutDataTypeStr=boolean
  Half adder1 : Subsystem
  Half adder2 : Subsystem
  Logical Operator1 : Logic  Operator=OR  AllPortsSameDT=off  OutDataTypeStr=boolean
  Out1 : Outport
  Out2 : Outport  Port=2
  wires:
  Logical Operator1/1 -> Out2/1
  In1/1 -> Half adder1/1(In1)
  Half adder2/1(Out1) -> Out1/1
  In2/1 -> Half adder1/2(In2)
  In3/1 -> Half adder2/2(In2)
  Half adder1/2(Out2) -> Logical Operator1/2
  Half adder1/1(Out1) -> Half adder2/1(In1)
  Half adder2/2(Out2) -> Logical Operator1/1

== system Multiplier/8-Bit_Multiplier/Full adder40 ==
  In1 : Inport  OutDataTypeStr=boolean
  In2 : Inport  Port=2  OutDataTypeStr=boolean
  In3 : Inport  Port=3  OutDataTypeStr=boolean
  Half adder1 : Subsystem
  Half adder2 : Subsystem
  Logical Operator1 : Logic  Operator=OR  AllPortsSameDT=off  OutDataTypeStr=boolean
  Out1 : Outport
  Out2 : Outport  Port=2
  wires:
  Logical Operator1/1 -> Out2/1
  In1/1 -> Half adder1/1(In1)
  Half adder2/1(Out1) -> Out1/1
  In2/1 -> Half adder1/2(In2)
  In3/1 -> Half adder2/2(In2)
  Half adder1/2(Out2) -> Logical Operator1/2
  Half adder1/1(Out1) -> Half adder2/1(In1)
  Half adder2/2(Out2) -> Logical Operator1/1

== system Multiplier/8-Bit_Multiplier/Full adder41 ==
  In1 : Inport  OutDataTypeStr=boolean
  In2 : Inport  Port=2  OutDataTypeStr=boolean
  In3 : Inport  Port=3  OutDataTypeStr=boolean
  Half adder1 : Subsystem
  Half adder2 : Subsystem
  Logical Operator1 : Logic  Operator=OR  AllPortsSameDT=off  OutDataTypeStr=boolean
  Out1 : Outport
  Out2 : Outport  Port=2
  wires:
  Logical Operator1/1 -> Out2/1
  In1/1 -> Half adder1/1(In1)
  Half adder2/1(Out1) -> Out1/1
  In2/1 -> Half adder1/2(In2)
  In3/1 -> Half adder2/2(In2)
  Half adder1/2(Out2) -> Logical Operator1/2
  Half adder1/1(Out1) -> Half adder2/1(In1)
  Half adder2/2(Out2) -> Logical Operator1/1

== system Multiplier/8-Bit_Multiplier/Full adder42 ==
  In1 : Inport  OutDataTypeStr=boolean
  In2 : Inport  Port=2  OutDataTypeStr=boolean
  In3 : Inport  Port=3  OutDataTypeStr=boolean
  Half adder1 : Subsystem
  Half adder2 : Subsystem
  Logical Operator1 : Logic  Operator=OR  AllPortsSameDT=off  OutDataTypeStr=boolean
  Out1 : Outport
  Out2 : Outport  Port=2
  wires:
  Logical Operator1/1 -> Out2/1
  In1/1 -> Half adder1/1(In1)
  Half adder2/1(Out1) -> Out1/1
  In2/1 -> Half adder1/2(In2)
  In3/1 -> Half adder2/2(In2)
  Half adder1/2(Out2) -> Logical Operator1/2
  Half adder1/1(Out1) -> Half adder2/1(In1)
  Half adder2/2(Out2) -> Logical Operator1/1

== system Multiplier/8-Bit_Multiplier/Full adder43 ==
  In1 : Inport  OutDataTypeStr=boolean
  In2 : Inport  Port=2  OutDataTypeStr=boolean
  In3 : Inport  Port=3  OutDataTypeStr=boolean
  Half adder1 : Subsystem
  Half adder2 : Subsystem
  Logical Operator1 : Logic  Operator=OR  AllPortsSameDT=off  OutDataTypeStr=boolean
  Out1 : Outport
  Out2 : Outport  Port=2
  wires:
  Logical Operator1/1 -> Out2/1
  In1/1 -> Half adder1/1(In1)
  Half adder2/1(Out1) -> Out1/1
  In2/1 -> Half adder1/2(In2)
  In3/1 -> Half adder2/2(In2)
  Half adder1/2(Out2) -> Logical Operator1/2
  Half adder1/1(Out1) -> Half adder2/1(In1)
  Half adder2/2(Out2) -> Logical Operator1/1

== system Multiplier/8-Bit_Multiplier/Full adder44 ==
  In1 : Inport  OutDataTypeStr=boolean
  In2 : Inport  Port=2  OutDataTypeStr=boolean
  In3 : Inport  Port=3  OutDataTypeStr=boolean
  Half adder1 : Subsystem
  Half adder2 : Subsystem
  Logical Operator1 : Logic  Operator=OR  AllPortsSameDT=off  OutDataTypeStr=boolean
  Out1 : Outport
  Out2 : Outport  Port=2
  wires:
  Logical Operator1/1 -> Out2/1
  In1/1 -> Half adder1/1(In1)
  Half adder2/1(Out1) -> Out1/1
  In2/1 -> Half adder1/2(In2)
  In3/1 -> Half adder2/2(In2)
  Half adder1/2(Out2) -> Logical Operator1/2
  Half adder1/1(Out1) -> Half adder2/1(In1)
  Half adder2/2(Out2) -> Logical Operator1/1

== system Multiplier/8-Bit_Multiplier/Full adder45 ==
  In1 : Inport  OutDataTypeStr=boolean
  In2 : Inport  Port=2  OutDataTypeStr=boolean
  In3 : Inport  Port=3  OutDataTypeStr=boolean
  Half adder1 : Subsystem
  Half adder2 : Subsystem
  Logical Operator1 : Logic  Operator=OR  AllPortsSameDT=off  OutDataTypeStr=boolean
  Out1 : Outport
  Out2 : Outport  Port=2
  wires:
  Logical Operator1/1 -> Out2/1
  In1/1 -> Half adder1/1(In1)
  Half adder2/1(Out1) -> Out1/1
  In2/1 -> Half adder1/2(In2)
  In3/1 -> Half adder2/2(In2)
  Half adder1/2(Out2) -> Logical Operator1/2
  Half adder1/1(Out1) -> Half adder2/1(In1)
  Half adder2/2(Out2) -> Logical Operator1/1

== system Multiplier/8-Bit_Multiplier/Full adder46 ==
  In1 : Inport  OutDataTypeStr=boolean
  In2 : Inport  Port=2  OutDataTypeStr=boolean
  In3 : Inport  Port=3  OutDataTypeStr=boolean
  Half adder1 : Subsystem
  Half adder2 : Subsystem
  Logical Operator1 : Logic  Operator=OR  AllPortsSameDT=off  OutDataTypeStr=boolean
  Out1 : Outport
  Out2 : Outport  Port=2
  wires:
  Logical Operator1/1 -> Out2/1
  In1/1 -> Half adder1/1(In1)
  Half adder2/1(Out1) -> Out1/1
  In2/1 -> Half adder1/2(In2)
  In3/1 -> Half adder2/2(In2)
  Half adder1/2(Out2) -> Logical Operator1/2
  Half adder1/1(Out1) -> Half adder2/1(In1)
  Half adder2/2(Out2) -> Logical Operator1/1

== system Multiplier/8-Bit_Multiplier/Full adder47 ==
  In1 : Inport  OutDataTypeStr=boolean
  In2 : Inport  Port=2  OutDataTypeStr=boolean
  In3 : Inport  Port=3  OutDataTypeStr=boolean
  Half adder1 : Subsystem
  Half adder2 : Subsystem
  Logical Operator1 : Logic  Operator=OR  AllPortsSameDT=off  OutDataTypeStr=boolean
  Out1 : Outport
  Out2 : Outport  Port=2
  wires:
  Logical Operator1/1 -> Out2/1
  In1/1 -> Half adder1/1(In1)
  Half adder2/1(Out1) -> Out1/1
  In2/1 -> Half adder1/2(In2)
  In3/1 -> Half adder2/2(In2)
  Half adder1/2(Out2) -> Logical Operator1/2
  Half adder1/1(Out1) -> Half adder2/1(In1)
  Half adder2/2(Out2) -> Logical Operator1/1

== system Multiplier/8-Bit_Multiplier/Full adder48 ==
  In1 : Inport  OutDataTypeStr=boolean
  In2 : Inport  Port=2  OutDataTypeStr=boolean
  In3 : Inport  Port=3  OutDataTypeStr=boolean
  Half adder1 : Subsystem
  Half adder2 : Subsystem
  Logical Operator1 : Logic  Operator=OR  AllPortsSameDT=off  OutDataTypeStr=boolean
  Out1 : Outport
  Out2 : Outport  Port=2
  wires:
  Logical Operator1/1 -> Out2/1
  In1/1 -> Half adder1/1(In1)
  Half adder2/1(Out1) -> Out1/1
  In2/1 -> Half adder1/2(In2)
  In3/1 -> Half adder2/2(In2)
  Half adder1/2(Out2) -> Logical Operator1/2
  Half adder1/1(Out1) -> Half adder2/1(In1)
  Half adder2/2(Out2) -> Logical Operator1/1

== system Multiplier/8-Bit_Multiplier/Full adder5 ==
  In1 : Inport  OutDataTypeStr=boolean
  In2 : Inport  Port=2  OutDataTypeStr=boolean
  In3 : Inport  Port=3  OutDataTypeStr=boolean
  Half adder1 : Subsystem
  Half adder2 : Subsystem
  Logical Operator1 : Logic  Operator=OR  AllPortsSameDT=off  OutDataTypeStr=boolean
  Out1 : Outport
  Out2 : Outport  Port=2
  wires:
  Logical Operator1/1 -> Out2/1
  In1/1 -> Half adder1/1(In1)
  Half adder2/1(Out1) -> Out1/1
  In2/1 -> Half adder1/2(In2)
  In3/1 -> Half adder2/2(In2)
  Half adder1/2(Out2) -> Logical Operator1/2
  Half adder1/1(Out1) -> Half adder2/1(In1)
  Half adder2/2(Out2) -> Logical Operator1/1

== system Multiplier/8-Bit_Multiplier/Full adder6 ==
  In1 : Inport  OutDataTypeStr=boolean
  In2 : Inport  Port=2  OutDataTypeStr=boolean
  In3 : Inport  Port=3  OutDataTypeStr=boolean
  Half adder1 : Subsystem
  Half adder2 : Subsystem
  Logical Operator1 : Logic  Operator=OR  AllPortsSameDT=off  OutDataTypeStr=boolean
  Out1 : Outport
  Out2 : Outport  Port=2
  wires:
  Logical Operator1/1 -> Out2/1
  In1/1 -> Half adder1/1(In1)
  Half adder2/1(Out1) -> Out1/1
  In2/1 -> Half adder1/2(In2)
  In3/1 -> Half adder2/2(In2)
  Half adder1/2(Out2) -> Logical Operator1/2
  Half adder1/1(Out1) -> Half adder2/1(In1)
  Half adder2/2(Out2) -> Logical Operator1/1

== system Multiplier/8-Bit_Multiplier/Full adder7 ==
  In1 : Inport  OutDataTypeStr=boolean
  In2 : Inport  Port=2  OutDataTypeStr=boolean
  In3 : Inport  Port=3  OutDataTypeStr=boolean
  Half adder1 : Subsystem
  Half adder2 : Subsystem
  Logical Operator1 : Logic  Operator=OR  AllPortsSameDT=off  OutDataTypeStr=boolean
  Out1 : Outport
  Out2 : Outport  Port=2
  wires:
  Logical Operator1/1 -> Out2/1
  In1/1 -> Half adder1/1(In1)
  Half adder2/1(Out1) -> Out1/1
  In2/1 -> Half adder1/2(In2)
  In3/1 -> Half adder2/2(In2)
  Half adder1/2(Out2) -> Logical Operator1/2
  Half adder1/1(Out1) -> Half adder2/1(In1)
  Half adder2/2(Out2) -> Logical Operator1/1

== system Multiplier/8-Bit_Multiplier/Full adder8 ==
  In1 : Inport  OutDataTypeStr=boolean
  In2 : Inport  Port=2  OutDataTypeStr=boolean
  In3 : Inport  Port=3  OutDataTypeStr=boolean
  Half adder1 : Subsystem
  Half adder2 : Subsystem
  Logical Operator1 : Logic  Operator=OR  AllPortsSameDT=off  OutDataTypeStr=boolean
  Out1 : Outport
  Out2 : Outport  Port=2
  wires:
  Logical Operator1/1 -> Out2/1
  In1/1 -> Half adder1/1(In1)
  Half adder2/1(Out1) -> Out1/1
  In2/1 -> Half adder1/2(In2)
  In3/1 -> Half adder2/2(In2)
  Half adder1/2(Out2) -> Logical Operator1/2
  Half adder1/1(Out1) -> Half adder2/1(In1)
  Half adder2/2(Out2) -> Logical Operator1/1

== system Multiplier/8-Bit_Multiplier/Full adder9 ==
  In1 : Inport  OutDataTypeStr=boolean
  In2 : Inport  Port=2  OutDataTypeStr=boolean
  In3 : Inport  Port=3  OutDataTypeStr=boolean
  Half adder1 : Subsystem
  Half adder2 : Subsystem
  Logical Operator1 : Logic  Operator=OR  AllPortsSameDT=off  OutDataTypeStr=boolean
  Out1 : Outport
  Out2 : Outport  Port=2
  wires:
  Logical Operator1/1 -> Out2/1
  In1/1 -> Half adder1/1(In1)
  Half adder2/1(Out1) -> Out1/1
  In2/1 -> Half adder1/2(In2)
  In3/1 -> Half adder2/2(In2)
  Half adder1/2(Out2) -> Logical Operator1/2
  Half adder1/1(Out1) -> Half adder2/1(In1)
  Half adder2/2(Out2) -> Logical Operator1/1

== system Multiplier/8-Bit_Multiplier/Half adder1 ==
  In1 : Inport  OutDataTypeStr=boolean
  In2 : Inport  Port=2  OutDataTypeStr=boolean
  Logical Operator : Logic  AllPortsSameDT=off  OutDataTypeStr=boolean
  Logical Operator1 : Logic  Operator=XOR  AllPortsSameDT=off  OutDataTypeStr=boolean
  Out1 : Outport
  Out2 : Outport  Port=2
  wires:
  In2/1 -> Logical Operator/2, Logical Operator1/2
  In1/1 -> Logical Operator/1, Logical Operator1/1
  Logical Operator1/1 -> Out1/1
  Logical Operator/1 -> Out2/1

== system Multiplier/8-Bit_Multiplier/Half adder2 ==
  In1 : Inport  OutDataTypeStr=boolean
  In2 : Inport  Port=2  OutDataTypeStr=boolean
  Logical Operator : Logic  AllPortsSameDT=off  OutDataTypeStr=boolean
  Logical Operator1 : Logic  Operator=XOR  AllPortsSameDT=off  OutDataTypeStr=boolean
  Out1 : Outport
  Out2 : Outport  Port=2
  wires:
  In2/1 -> Logical Operator/2, Logical Operator1/2
  In1/1 -> Logical Operator/1, Logical Operator1/1
  Logical Operator1/1 -> Out1/1
  Logical Operator/1 -> Out2/1

== system Multiplier/8-Bit_Multiplier/Half adder3 ==
  In1 : Inport  OutDataTypeStr=boolean
  In2 : Inport  Port=2  OutDataTypeStr=boolean
  Logical Operator : Logic  AllPortsSameDT=off  OutDataTypeStr=boolean
  Logical Operator1 : Logic  Operator=XOR  AllPortsSameDT=off  OutDataTypeStr=boolean
  Out1 : Outport
  Out2 : Outport  Port=2
  wires:
  In2/1 -> Logical Operator/2, Logical Operator1/2
  In1/1 -> Logical Operator/1, Logical Operator1/1
  Logical Operator1/1 -> Out1/1
  Logical Operator/1 -> Out2/1

== system Multiplier/8-Bit_Multiplier/Half adder4 ==
  In1 : Inport  OutDataTypeStr=boolean
  In2 : Inport  Port=2  OutDataTypeStr=boolean
  Logical Operator : Logic  AllPortsSameDT=off  OutDataTypeStr=boolean
  Logical Operator1 : Logic  Operator=XOR  AllPortsSameDT=off  OutDataTypeStr=boolean
  Out1 : Outport
  Out2 : Outport  Port=2
  wires:
  In2/1 -> Logical Operator/2, Logical Operator1/2
  In1/1 -> Logical Operator/1, Logical Operator1/1
  Logical Operator1/1 -> Out1/1
  Logical Operator/1 -> Out2/1

== system Multiplier/8-Bit_Multiplier/Half adder5 ==
  In1 : Inport  OutDataTypeStr=boolean
  In2 : Inport  Port=2  OutDataTypeStr=boolean
  Logical Operator : Logic  AllPortsSameDT=off  OutDataTypeStr=boolean
  Logical Operator1 : Logic  Operator=XOR  AllPortsSameDT=off  OutDataTypeStr=boolean
  Out1 : Outport
  Out2 : Outport  Port=2
  wires:
  In2/1 -> Logical Operator/2, Logical Operator1/2
  In1/1 -> Logical Operator/1, Logical Operator1/1
  Logical Operator1/1 -> Out1/1
  Logical Operator/1 -> Out2/1

== system Multiplier/8-Bit_Multiplier/Half adder6 ==
  In1 : Inport  OutDataTypeStr=boolean
  In2 : Inport  Port=2  OutDataTypeStr=boolean
  Logical Operator : Logic  AllPortsSameDT=off  OutDataTypeStr=boolean
  Logical Operator1 : Logic  Operator=XOR  AllPortsSameDT=off  OutDataTypeStr=boolean
  Out1 : Outport
  Out2 : Outport  Port=2
  wires:
  In2/1 -> Logical Operator/2, Logical Operator1/2
  In1/1 -> Logical Operator/1, Logical Operator1/1
  Logical Operator1/1 -> Out1/1
  Logical Operator/1 -> Out2/1

== system Multiplier/8-Bit_Multiplier/Half adder7 ==
  In1 : Inport  OutDataTypeStr=boolean
  In2 : Inport  Port=2  OutDataTypeStr=boolean
  Logical Operator : Logic  AllPortsSameDT=off  OutDataTypeStr=boolean
  Logical Operator1 : Logic  Operator=XOR  AllPortsSameDT=off  OutDataTypeStr=boolean
  Out1 : Outport
  Out2 : Outport  Port=2
  wires:
  In2/1 -> Logical Operator/2, Logical Operator1/2
  In1/1 -> Logical Operator/1, Logical Operator1/1
  Logical Operator1/1 -> Out1/1
  Logical Operator/1 -> Out2/1

== system Multiplier/8-Bit_Multiplier/Half adder8 ==
  In1 : Inport  OutDataTypeStr=boolean
  In2 : Inport  Port=2  OutDataTypeStr=boolean
  Logical Operator : Logic  AllPortsSameDT=off  OutDataTypeStr=boolean
  Logical Operator1 : Logic  Operator=XOR  AllPortsSameDT=off  OutDataTypeStr=boolean
  Out1 : Outport
  Out2 : Outport  Port=2
  wires:
  In2/1 -> Logical Operator/2, Logical Operator1/2
  In1/1 -> Logical Operator/1, Logical Operator1/1
  Logical Operator1/1 -> Out1/1
  Logical Operator/1 -> Out2/1

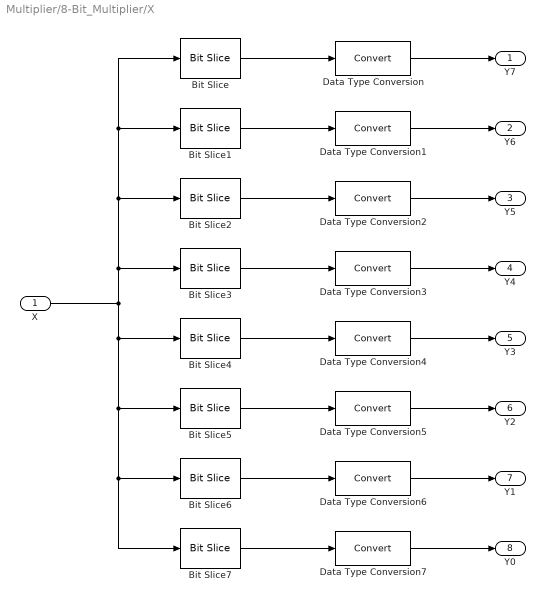
== system Multiplier/8-Bit_Multiplier/X ==
  X : Inport  OutDataTypeStr=uint8  SampleTime=1
  Bit Slice : hdlsllib/Logic and Bit Operations/Bit Slice  lidx=7  ridx=7
      settings: SourceProductName=Simulink  SourceProductBaseCode=SL
  Bit Slice1 : hdlsllib/Logic and Bit Operations/Bit Slice  lidx=6  ridx=6
      settings: SourceProductName=Simulink  SourceProductBaseCode=SL
  Bit Slice2 : hdlsllib/Logic and Bit Operations/Bit Slice  lidx=5  ridx=5
      settings: SourceProductName=Simulink  SourceProductBaseCode=SL
  Bit Slice3 : hdlsllib/Logic and Bit Operations/Bit Slice  lidx=4  ridx=4
      settings: SourceProductName=Simulink  SourceProductBaseCode=SL
  Bit Slice4 : hdlsllib/Logic and Bit Operations/Bit Slice  lidx=3  ridx=3
      settings: SourceProductName=Simulink  SourceProductBaseCode=SL
  Bit Slice5 : hdlsllib/Logic and Bit Operations/Bit Slice  lidx=2  ridx=2
      settings: SourceProductName=Simulink  SourceProductBaseCode=SL
  Bit Slice6 : hdlsllib/Logic and Bit Operations/Bit Slice  lidx=1  ridx=1
      settings: SourceProductName=Simulink  SourceProductBaseCode=SL
  Bit Slice7 : hdlsllib/Logic and Bit Operations/Bit Slice  lidx=0  ridx=0
      settings: SourceProductName=Simulink  SourceProductBaseCode=SL
  Data Type Conversion{,1..7} (8 alike) : DataTypeConversion
  Y7 : Outport
  Y6 : Outport  Port=2
  Y5 : Outport  Port=3
  Y4 : Outport  Port=4
  Y3 : Outport  Port=5
  Y2 : Outport  Port=6
  Y1 : Outport  Port=7
  Y0 : Outport  Port=8
  wires:
  Bit Slice6/1 -> Data Type Conversion6/1
  X/1 -> Bit Slice3/1, Bit Slice2/1, Bit Slice1/1, Bit Slice/1, Bit Slice4/1, Bit Slice5/1, Bit Slice6/1, Bit Slice7/1
  Bit Slice/1 -> Data Type Conversion/1
  Bit Slice7/1 -> Data Type Conversion7/1
  Bit Slice4/1 -> Data Type Conversion4/1
  Bit Slice1/1 -> Data Type Conversion1/1
  Bit Slice3/1 -> Data Type Conversion3/1
  Data Type Conversion1/1 -> Y6/1
  Data Type Conversion7/1 -> Y0/1
  Data Type Conversion5/1 -> Y2/1
  Data Type Conversion3/1 -> Y4/1
  Data Type Conversion4/1 -> Y3/1
  Bit Slice2/1 -> Data Type Conversion2/1
  Bit Slice5/1 -> Data Type Conversion5/1
  Data Type Conversion6/1 -> Y1/1
  Data Type Conversion/1 -> Y7/1
  Data Type Conversion2/1 -> Y5/1
